simulink library "MBDS_Applications"  (R2018b)
settings: Solver=ode45  StartTime=0.0  StopTime=10.0  RelTol=1e-3
undefined symbols (not defined in the file or in its folder): Ts
libraries: KIBES_Signal x297, simulink x7
(part 6 of 6)

== system MBDS_Applications/APP_MyApplication/DTC/GetBit3/LoopOverBits ==
  note: No saturation
      | needed !
  note: Determine bit value
  note: Generate bit mask
  u : Inport
  SEL : Inport  Port=2
  Assignment1 : Assignment  IndexMode=Zero-based  IndexOptions=Index vector (port)  Indices=1  OutputSizes=[1 1]
  Bitwise Operator1 : simulink/Logic and Bit Operations/Bitwise Operator  logicop=AND  UseBitMask=off  NumInputPorts=2  BitMask=bin2dec('11011001')  BitMaskRealWorld=Stored Integer
  Constant2 : Constant  Value=0  OutDataTypeStr=Inherit: Inherit via back propagation
  Constant3 : Constant  OutDataTypeStr=Inherit: Inherit via back propagation
  Data Type Duplicate : DataTypeDuplicate  InitFcn=|
      | try
      |    MBDS_BlockCallback('Update', gcb);
      | end
  DataType : DataTypeConversion  OutDataTypeStr=boolean
  DataType1 : DataTypeConversion  OutDataTypeStr=uint8
  For Iterator : ForIterator  IterationSource=external  IndexMode=Zero-based  IterationVariableDataType=int8
  IndexOffset : Constant  Value=0  OutDataTypeStr=Inherit: Inherit via back propagation
  Relational Operator : RelationalOperator  Operator=~=  OutDataTypeStr=boolean  RndMeth=Nearest
  Selector : Selector  IndexMode=Zero-based  IndexOptions=Index vector (port)  Indices=[1 3]  OutputSizes=1
  Shift Arithmetic : ArithShift  BitShiftNumberSource=Input port  BitShiftNumber=8  BitShiftDirection=Left
      settings: InputPortMap=u0,p1
  Subtract : Sum  Inputs=+-  OutDataTypeStr=Inherit: Inherit via back propagation  InputSameDT=on
  Width : Width  DataType=uint8
  y : Outport
  wires:
  u/1 -> Data Type Duplicate/1, Bitwise Operator1/1
  DataType1/1 -> Selector/1
  SEL/1 -> Width/1, DataType/1, DataType1/1
  DataType/1 -> Assignment1/1
  Assignment1/1 -> y/1
  Relational Operator/1 -> Assignment1/2
  Constant2/1 -> Relational Operator/2
  Bitwise Operator1/1 -> Relational Operator/1
  Shift Arithmetic/1 -> Bitwise Operator1/2
  Constant3/1 -> Data Type Duplicate/2, Shift Arithmetic/1
  Width/1 -> For Iterator/1
  For Iterator/1 -> Assignment1/3, Selector/2
  Selector/1 -> Subtract/1
  Subtract/1 -> Shift Arithmetic/2
  IndexOffset/1 -> Subtract/2

== system MBDS_Applications/APP_MyApplication/DTC/GetBit4/LoopOverBits ==
  note: No saturation
      | needed !
  note: Determine bit value
  note: Generate bit mask
  u : Inport
  SEL : Inport  Port=2
  Assignment1 : Assignment  IndexMode=Zero-based  IndexOptions=Index vector (port)  Indices=1  OutputSizes=[1 1]
  Bitwise Operator1 : simulink/Logic and Bit Operations/Bitwise Operator  logicop=AND  UseBitMask=off  NumInputPorts=2  BitMask=bin2dec('11011001')  BitMaskRealWorld=Stored Integer
  Constant2 : Constant  Value=0  OutDataTypeStr=Inherit: Inherit via back propagation
  Constant3 : Constant  OutDataTypeStr=Inherit: Inherit via back propagation
  Data Type Duplicate : DataTypeDuplicate  InitFcn=|
      | try
      |    MBDS_BlockCallback('Update', gcb);
      | end
  DataType : DataTypeConversion  OutDataTypeStr=boolean
  DataType1 : DataTypeConversion  OutDataTypeStr=uint8
  For Iterator : ForIterator  IterationSource=external  IndexMode=Zero-based  IterationVariableDataType=int8
  IndexOffset : Constant  Value=0  OutDataTypeStr=Inherit: Inherit via back propagation
  Relational Operator : RelationalOperator  Operator=~=  OutDataTypeStr=boolean  RndMeth=Nearest
  Selector : Selector  IndexMode=Zero-based  IndexOptions=Index vector (port)  Indices=[1 3]  OutputSizes=1
  Shift Arithmetic : ArithShift  BitShiftNumberSource=Input port  BitShiftNumber=8  BitShiftDirection=Left
      settings: InputPortMap=u0,p1
  Subtract : Sum  Inputs=+-  OutDataTypeStr=Inherit: Inherit via back propagation  InputSameDT=on
  Width : Width  DataType=uint8
  y : Outport
  wires:
  u/1 -> Data Type Duplicate/1, Bitwise Operator1/1
  DataType1/1 -> Selector/1
  SEL/1 -> Width/1, DataType/1, DataType1/1
  DataType/1 -> Assignment1/1
  Assignment1/1 -> y/1
  Relational Operator/1 -> Assignment1/2
  Constant2/1 -> Relational Operator/2
  Bitwise Operator1/1 -> Relational Operator/1
  Shift Arithmetic/1 -> Bitwise Operator1/2
  Constant3/1 -> Data Type Duplicate/2, Shift Arithmetic/1
  Width/1 -> For Iterator/1
  For Iterator/1 -> Assignment1/3, Selector/2
  Selector/1 -> Subtract/1
  Subtract/1 -> Shift Arithmetic/2
  IndexOffset/1 -> Subtract/2

== system MBDS_Applications/APP_MyApplication/DTC/GetBit5/LoopOverBits ==
  note: No saturation
      | needed !
  note: Determine bit value
  note: Generate bit mask
  u : Inport
  SEL : Inport  Port=2
  Assignment1 : Assignment  IndexMode=Zero-based  IndexOptions=Index vector (port)  Indices=1  OutputSizes=[1 1]
  Bitwise Operator1 : simulink/Logic and Bit Operations/Bitwise Operator  logicop=AND  UseBitMask=off  NumInputPorts=2  BitMask=bin2dec('11011001')  BitMaskRealWorld=Stored Integer
  Constant2 : Constant  Value=0  OutDataTypeStr=Inherit: Inherit via back propagation
  Constant3 : Constant  OutDataTypeStr=Inherit: Inherit via back propagation
  Data Type Duplicate : DataTypeDuplicate  InitFcn=|
      | try
      |    MBDS_BlockCallback('Update', gcb);
      | end
  DataType : DataTypeConversion  OutDataTypeStr=boolean
  DataType1 : DataTypeConversion  OutDataTypeStr=uint8
  For Iterator : ForIterator  IterationSource=external  IndexMode=Zero-based  IterationVariableDataType=int8
  IndexOffset : Constant  Value=0  OutDataTypeStr=Inherit: Inherit via back propagation
  Relational Operator : RelationalOperator  Operator=~=  OutDataTypeStr=boolean  RndMeth=Nearest
  Selector : Selector  IndexMode=Zero-based  IndexOptions=Index vector (port)  Indices=[1 3]  OutputSizes=1
  Shift Arithmetic : ArithShift  BitShiftNumberSource=Input port  BitShiftNumber=8  BitShiftDirection=Left
      settings: InputPortMap=u0,p1
  Subtract : Sum  Inputs=+-  OutDataTypeStr=Inherit: Inherit via back propagation  InputSameDT=on
  Width : Width  DataType=uint8
  y : Outport
  wires:
  u/1 -> Data Type Duplicate/1, Bitwise Operator1/1
  DataType1/1 -> Selector/1
  SEL/1 -> Width/1, DataType/1, DataType1/1
  DataType/1 -> Assignment1/1
  Assignment1/1 -> y/1
  Relational Operator/1 -> Assignment1/2
  Constant2/1 -> Relational Operator/2
  Bitwise Operator1/1 -> Relational Operator/1
  Shift Arithmetic/1 -> Bitwise Operator1/2
  Constant3/1 -> Data Type Duplicate/2, Shift Arithmetic/1
  Width/1 -> For Iterator/1
  For Iterator/1 -> Assignment1/3, Selector/2
  Selector/1 -> Subtract/1
  Subtract/1 -> Shift Arithmetic/2
  IndexOffset/1 -> Subtract/2

== system MBDS_Applications/APP_MyApplication/DTC/GetBit6/LoopOverBits ==
  note: No saturation
      | needed !
  note: Determine bit value
  note: Generate bit mask
  u : Inport
  SEL : Inport  Port=2
  Assignment1 : Assignment  IndexMode=Zero-based  IndexOptions=Index vector (port)  Indices=1  OutputSizes=[1 1]
  Bitwise Operator1 : simulink/Logic and Bit Operations/Bitwise Operator  logicop=AND  UseBitMask=off  NumInputPorts=2  BitMask=bin2dec('11011001')  BitMaskRealWorld=Stored Integer
  Constant2 : Constant  Value=0  OutDataTypeStr=Inherit: Inherit via back propagation
  Constant3 : Constant  OutDataTypeStr=Inherit: Inherit via back propagation
  Data Type Duplicate : DataTypeDuplicate  InitFcn=|
      | try
      |    MBDS_BlockCallback('Update', gcb);
      | end
  DataType : DataTypeConversion  OutDataTypeStr=boolean
  DataType1 : DataTypeConversion  OutDataTypeStr=uint8
  For Iterator : ForIterator  IterationSource=external  IndexMode=Zero-based  IterationVariableDataType=int8
  IndexOffset : Constant  Value=0  OutDataTypeStr=Inherit: Inherit via back propagation
  Relational Operator : RelationalOperator  Operator=~=  OutDataTypeStr=boolean  RndMeth=Nearest
  Selector : Selector  IndexMode=Zero-based  IndexOptions=Index vector (port)  Indices=[1 3]  OutputSizes=1
  Shift Arithmetic : ArithShift  BitShiftNumberSource=Input port  BitShiftNumber=8  BitShiftDirection=Left
      settings: InputPortMap=u0,p1
  Subtract : Sum  Inputs=+-  OutDataTypeStr=Inherit: Inherit via back propagation  InputSameDT=on
  Width : Width  DataType=uint8
  y : Outport
  wires:
  u/1 -> Data Type Duplicate/1, Bitwise Operator1/1
  DataType1/1 -> Selector/1
  SEL/1 -> Width/1, DataType/1, DataType1/1
  DataType/1 -> Assignment1/1
  Assignment1/1 -> y/1
  Relational Operator/1 -> Assignment1/2
  Constant2/1 -> Relational Operator/2
  Bitwise Operator1/1 -> Relational Operator/1
  Shift Arithmetic/1 -> Bitwise Operator1/2
  Constant3/1 -> Data Type Duplicate/2, Shift Arithmetic/1
  Width/1 -> For Iterator/1
  For Iterator/1 -> Assignment1/3, Selector/2
  Selector/1 -> Subtract/1
  Subtract/1 -> Shift Arithmetic/2
  IndexOffset/1 -> Subtract/2

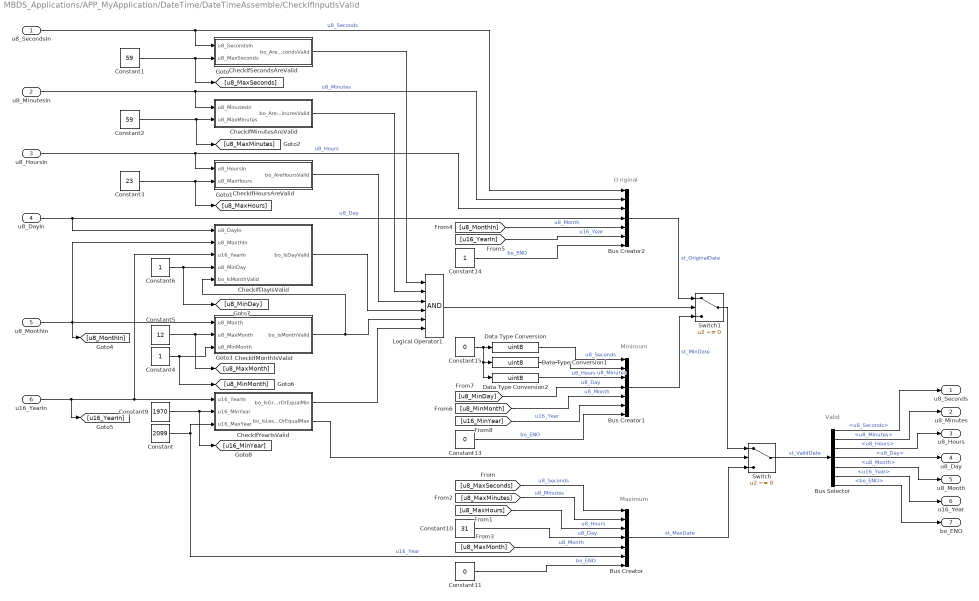
== system MBDS_Applications/APP_MyApplication/DateTime/DateTimeAssemble/CheckIfInputIsValid ==
  note: Maximum
  note: Minimum
  note: O riginal
  note: Valid
  u8_SecondsIn : Inport  OutDataTypeStr=uint8
  u8_MinutesIn : Inport  Port=2  OutDataTypeStr=uint8
  u8_HoursIn : Inport  Port=3  OutDataTypeStr=uint8
  u8_DayIn : Inport  Port=4  OutDataTypeStr=uint8
  u8_MonthIn : Inport  Port=5  OutDataTypeStr=uint8
  u16_YearIn : Inport  Port=6  OutDataTypeStr=uint16
  Bus Creator : BusCreator  Inputs='u8_Seconds','u8_Minutes','u8_Hours','u8_Day','u8_Month','u16_Year','bo_ENO'
  Bus Creator1 : BusCreator  Inputs='u8_Seconds','u8_Minutes','u8_Hours','u8_Day','u8_Month','u16_Year','bo_ENO'
  Bus Creator2 : BusCreator  Inputs='u8_Seconds','u8_Minutes','u8_Hours','u8_Day','u8_Month','u16_Year','bo_ENO'
  Bus Selector : BusSelector  OutputSignals=u8_Seconds,u8_Minutes,u8_Hours,u8_Day,u8_Month,u16_Year,bo_ENO
  CheckIfDayIsValid : Subsystem
  CheckIfHoursAreValid : Subsystem
  CheckIfMinutesAreValid : Subsystem
  CheckIfMonthIsValid : Subsystem
  CheckIfSecondsAreValid : Subsystem
  CheckIfYearIsValid : Subsystem
  Constant : Constant  Value=2099  OutDataTypeStr=uint16
  Constant1 : Constant  Value=59  OutDataTypeStr=uint8
  Constant10 : Constant  Value=31  OutDataTypeStr=uint8
  Constant11 : Constant  Value=0  OutDataTypeStr=boolean
  Constant13 : Constant  Value=0  OutDataTypeStr=boolean
  Constant14 : Constant  OutDataTypeStr=boolean
  Constant15 : Constant  Value=0  OutDataTypeStr=uint8
  Constant2 : Constant  Value=59  OutDataTypeStr=uint8
  Constant3 : Constant  Value=23  OutDataTypeStr=uint8
  Constant4 : Constant  OutDataTypeStr=uint8
  Constant5 : Constant  Value=12  OutDataTypeStr=uint8
  Constant6 : Constant  OutDataTypeStr=uint8
  Constant9 : Constant  Value=1970  OutDataTypeStr=uint16
  Data Type Conversion : DataTypeConversion  OutDataTypeStr=uint8
  Data Type Conversion1 : DataTypeConversion  OutDataTypeStr=uint8
  Data Type Conversion2 : DataTypeConversion  OutDataTypeStr=uint8
  Logical Operator1 : Logic  Inputs=6  AllPortsSameDT=off  OutDataTypeStr=boolean
  Switch : Switch  Criteria=u2 ~= 0
  Switch1 : Switch  Criteria=u2 ~= 0
  u8_Seconds : Outport  OutDataTypeStr=uint8
  u8_Minutes : Outport  Port=2  OutDataTypeStr=uint8
  u8_Hours : Outport  Port=3  OutDataTypeStr=uint8
  u8_Day : Outport  Port=4  OutDataTypeStr=uint8
  u8_Month : Outport  Port=5  OutDataTypeStr=uint8
  u16_Year : Outport  Port=6  OutDataTypeStr=uint16
  bo_ENO : Outport  Port=7  OutDataTypeStr=boolean
  wires:
  Data Type Conversion2/1 -> Bus Creator1/3  "u8_Hours"
  Data Type Conversion1/1 -> Bus Creator1/2  "u8_Minutes"
  [u16_MinYear] -> Bus Creator1/6  "u16_Year"
  Constant6/1 -> CheckIfDayIsValid/4(u8_MinDay), [u8_MinDay]
  Constant4/1 -> CheckIfMonthIsValid/3(u8_MinMonth), [u8_MinMonth]
  CheckIfYearIsValid/2(bo_IsLessOrEqualMax) -> Switch/2
  CheckIfYearIsValid/1(bo_IsGreaterOrEqualMin) -> Logical Operator1/6
  CheckIfMonthIsValid/1(bo_IsMonthValid) -> Logical Operator1/5, CheckIfDayIsValid/5(bo_IsMonthValid)
  Constant2/1 -> CheckIfMinutesAreValid/2(u8_MaxMinutes), [u8_MaxMinutes]
  CheckIfSecondsAreValid/1(bo_AreSecondsValid) -> Logical Operator1/1
  Constant1/1 -> CheckIfSecondsAreValid/2(u8_MaxSeconds), [u8_MaxSeconds]
  CheckIfDayIsValid/1(bo_IsDayValid) -> Logical Operator1/4
  u8_MonthIn/1 -> CheckIfMonthIsValid/1(u8_Month), [u8_MonthIn], CheckIfDayIsValid/2(u8_MonthIn)
  Bus Selector/5 -> u8_Month/1  "<u8_Month>"
  [u8_MaxSeconds] -> Bus Creator/1  "u8_Seconds"
  Constant15/1 -> Data Type Conversion/1, Data Type Conversion1/1, Data Type Conversion2/1
  [u8_MinDay] -> Bus Creator1/4  "u8_Day"
  Data Type Conversion/1 -> Bus Creator1/1  "u8_Seconds"
  Constant14/1 -> Bus Creator2/7  "bo_ENO"
  Switch/1 -> Bus Selector/1  "st_ValidDate"
  Bus Creator/1 -> Switch/3  "st_MaxDate"
  Switch1/1 -> Switch/1
  Bus Creator2/1 -> Switch1/1  "st_OriginalDate"
  Bus Selector/7 -> bo_ENO/1  "<bo_ENO>"
  Bus Selector/6 -> u16_Year/1  "<u16_Year>"
  Bus Selector/1 -> u8_Seconds/1  "<u8_Seconds>"
  Bus Selector/2 -> u8_Minutes/1  "<u8_Minutes>"
  Bus Selector/3 -> u8_Hours/1  "<u8_Hours>"
  Bus Selector/4 -> u8_Day/1  "<u8_Day>"
  Constant13/1 -> Bus Creator1/7  "bo_ENO"
  [u16_YearIn] -> Bus Creator2/6  "u16_Year"
  [u8_MonthIn] -> Bus Creator2/5  "u8_Month"
  Bus Creator1/1 -> Switch1/3  "st_MinDate"
  Logical Operator1/1 -> Switch1/2
  [u8_MinMonth] -> Bus Creator1/5  "u8_Month"
  [u8_MaxMonth] -> Bus Creator/5  "u8_Month"
  Constant10/1 -> Bus Creator/4  "u8_Day"
  Constant3/1 -> [u8_MaxHours], CheckIfHoursAreValid/2(u8_MaxHours)
  [u8_MaxHours] -> Bus Creator/3  "u8_Hours"
  [u8_MaxMinutes] -> Bus Creator/2  "u8_Minutes"
  Constant11/1 -> Bus Creator/7  "bo_ENO"
  Constant9/1 -> CheckIfYearIsValid/2(u16_MinYear), [u16_MinYear]
  CheckIfHoursAreValid/1(bo_AreHoursValid) -> Logical Operator1/3
  CheckIfMinutesAreValid/1(bo_AreMinutesValid) -> Logical Operator1/2
  Constant5/1 -> [u8_MaxMonth], CheckIfMonthIsValid/2(u8_MaxMonth)
  u8_DayIn/1 -> CheckIfDayIsValid/1(u8_DayIn), Bus Creator2/4  "u8_Day"
  u8_SecondsIn/1 -> Bus Creator2/1, CheckIfSecondsAreValid/1(u8_SecondsIn)  "u8_Seconds"
  u8_MinutesIn/1 -> CheckIfMinutesAreValid/1(u8_MinutesIn), Bus Creator2/2  "u8_Minutes"
  u8_HoursIn/1 -> CheckIfHoursAreValid/1(u8_HoursIn), Bus Creator2/3  "u8_Hours"
  Constant/1 -> CheckIfYearIsValid/3(u16_MaxYear), Bus Creator/6  "u16_Year"
  u16_YearIn/1 -> [u16_YearIn], CheckIfDayIsValid/3(u16_YearIn), CheckIfYearIsValid/1(u16_YearIn)

== system MBDS_Applications/APP_MyApplication/DateTime/DateTimeAssemble/ConvertToDateTime ==
  u8_Seconds : Inport  OutDataTypeStr=uint8
  u8_Minutes : Inport  Port=2  OutDataTypeStr=uint8
  u8_Hours : Inport  Port=3  OutDataTypeStr=uint8
  u16_NrOfDays : Inport  Port=4  OutDataTypeStr=uint16
  Add : Sum  Inputs=++++  OutDataTypeStr=uint32
  ConvertDaysToSeconds : Subsystem
  ConvertHoursToSeconds : Subsystem
  ConvertMinutesToSeconds : Subsystem
  u32_DateTime : Outport  OutDataTypeStr=uint32
  wires:
  u16_NrOfDays/1 -> ConvertDaysToSeconds/1(u16_NrOfDays)
  u8_Hours/1 -> ConvertHoursToSeconds/1(u8_Hours)
  u8_Minutes/1 -> ConvertMinutesToSeconds/1(u8_Minutes)
  ConvertDaysToSeconds/1(u32_SecFromDays) -> Add/4
  ConvertHoursToSeconds/1(u32_SecFromHrs) -> Add/3
  ConvertMinutesToSeconds/1(u16_SecFromMins) -> Add/2
  Add/1 -> u32_DateTime/1
  u8_Seconds/1 -> Add/1

== system MBDS_Applications/APP_MyApplication/DateTime/DateTimeAssemble/ConvertToNrOfDays ==
  note: Convert to number of days
  u8_Day : Inport  OutDataTypeStr=uint8
  u8_Month : Inport  Port=2  OutDataTypeStr=uint8
  u16_Year : Inport  Port=3  OutDataTypeStr=uint16
  AddDays : Subsystem
  AddDaysForCompleteMonths : Subsystem  TreatAsAtomicUnit=on
  AddDaysForCompleteYears : Subsystem
  CheckIfDateInLeapYearBeforeMarch : Subsystem
  Subtract2 : Sum  Inputs=+++-  OutDataTypeStr=uint16
  u16_NrOfDays : Outport  OutDataTypeStr=uint16
  wires:
  CheckIfDateInLeapYearBeforeMarch/1(bo_MinusOne) -> Subtract2/4
  AddDaysForCompleteYears/1(u16_DaysForYears) -> Subtract2/3
  AddDays/1(u8_CompleteDays) -> Subtract2/1
  AddDaysForCompleteMonths/1(u16_DaysForMonths) -> Subtract2/2
  u8_Day/1 -> AddDays/1(u8_Day)
  u8_Month/1 -> AddDaysForCompleteMonths/1(u8_Month), CheckIfDateInLeapYearBeforeMarch/1(u8_Month)
  Subtract2/1 -> u16_NrOfDays/1
  u16_Year/1 -> AddDaysForCompleteYears/1(u16_Year), CheckIfDateInLeapYearBeforeMarch/2(u16_Year)

== system MBDS_Applications/APP_MyApplication/DateTime/DateTimeDisassemble/CheckIfTimeDataIsValid ==
  note: Check if time data is valid
  note: 2099-12-31-23:59:59
  u32_DateTime : Inport  OutDataTypeStr=uint32
  Constant14 : Constant  Value=4102444799  OutDataTypeStr=uint32
  Relational Operator : RelationalOperator  Operator=<=  OutDataTypeStr=boolean  RndMeth=Nearest
  bo_ENO : Outport  OutDataTypeStr=boolean
  wires:
  Relational Operator/1 -> bo_ENO/1
  u32_DateTime/1 -> Relational Operator/1
  Constant14/1 -> Relational Operator/2

== system MBDS_Applications/APP_MyApplication/DateTime/DateTimeDisassemble/CheckLeapYearsAndRemainingDays ==
  note: avoid overflow
  note: Check leap year and calculate remaining days in current year
  note: Year
  u16_NrOfDays : Inport  OutDataTypeStr=uint16
  Add3 : Sum  Inputs=++-  OutDataTypeStr=uint16
  CalculateLeapYearsSince1970 : Subsystem
  CalculateRemainingDays : Subsystem
  CheckIfCorrectedTempYearIsLeap : Subsystem
  CheckIfTempYearIsCorrect : Subsystem
  CheckLeapYear : Subsystem
  Constant2 : Constant  OutDataTypeStr=uint16
  Constant6 : Constant  Value=0  OutDataTypeStr=uint16
  DaysPerNonLeapYear : Constant  Value=365  OutDataTypeStr=uint16
  Math Function3 : Math  Operator=rem  OutputSignalType=real  SaturateOnIntegerOverflow=on
  Relational Operator1 : RelationalOperator  Operator===  OutDataTypeStr=boolean  RndMeth=Nearest  InputSameDT=on
  Switch1 : Switch  Criteria=u2 ~= 0  OutDataTypeStr=uint16
  u16_TempDate : Outport  OutDataTypeStr=uint16
  u16_Year : Outport  Port=2  OutDataTypeStr=uint16
  bo_LeapYear : Outport  Port=3  OutDataTypeStr=boolean
  wires:
  [u16_NrOfLeapYears] -> CalculateRemainingDays/4(u16_NrOfLeapYears)
  CheckIfCorrectedTempYearIsLeap/1(bo_IsCorrectedYearLeapYear) -> CalculateRemainingDays/1(bo_IsCorrectedYearLeapYear)
  CalculateRemainingDays/1(u16_TempDate) -> u16_TempDate/1
  CheckIfTempYearIsCorrect/1(bo_IsTempYearCorrect) -> CalculateRemainingDays/2(bo_IsTempYearCorrect), Switch1/2
  [u16_NrOfLeapYears] -> CheckIfTempYearIsCorrect/2(u16_NrOfLeapYears)
  CalculateLeapYearsSince1970/1(u16_NrOfLeapYears) -> [u16_NrOfLeapYears]
  Relational Operator1/1 -> Add3/1
  Constant2/1 -> Add3/3
  Constant6/1 -> Relational Operator1/1
  CheckLeapYear/1(bo_LeapYear) -> bo_LeapYear/1
  Add3/1 -> CheckIfCorrectedTempYearIsLeap/1(u16_CorrectedTempYear), Switch1/3
  CalculateLeapYearsSince1970/2(u16_TempYear) -> Relational Operator1/2, Add3/2, Switch1/1
  Switch1/1 -> u16_Year/1, CheckLeapYear/1(u16_Year)
  Math Function3/1 -> CheckIfTempYearIsCorrect/1(u16_TempRemainingDays), CalculateRemainingDays/3(u16_TempRemainingDays)
  DaysPerNonLeapYear/1 -> CalculateLeapYearsSince1970/2(u16_DaysPerCommonYear), Math Function3/2, CalculateRemainingDays/5(u16_DaysPerCommonYear)
  u16_NrOfDays/1 -> Math Function3/1, CalculateLeapYearsSince1970/1(u16_NrOfDays)

== system MBDS_Applications/APP_MyApplication/DateTime/DateTimeDisassemble/ConvertToDayOfWeek ==
  note: Convert to day of week
  note: 1970-01-01 is Thursday
  u16_NrOfDays : Inport  OutDataTypeStr=uint16
  Add2 : Sum  OutDataTypeStr=uint16
  Add3 : Sum  OutDataTypeStr=uint16
  Constant3 : Constant  Value=7  OutDataTypeStr=uint16
  Constant4 : Constant  Value=3  OutDataTypeStr=uint8
  Constant5 : Constant  OutDataTypeStr=uint8
  Data Type Conversion3 : DataTypeConversion  OutDataTypeStr=uint8
  Math Function : Math  Operator=rem  OutputSignalType=real  SaturateOnIntegerOverflow=on
  u8_DayOfWeek : Outport  OutDataTypeStr=uint8
  wires:
  u16_NrOfDays/1 -> Add2/1
  Add3/1 -> Data Type Conversion3/1
  Math Function/1 -> Add3/1
  Add2/1 -> Math Function/1
  Constant4/1 -> Add2/2
  Constant3/1 -> Math Function/2
  Constant5/1 -> Add3/2
  Data Type Conversion3/1 -> u8_DayOfWeek/1

== system MBDS_Applications/APP_MyApplication/DateTime/DateTimeDisassemble/ConvertToMonthAndDay ==
  note: Convert to month and day
  note: Check if there are less days remaining than the next month has
  note: Count number of cycles (= Month - 1)
  note: Days per month
  u16_TempDate : Inport  OutDataTypeStr=uint16
  bo_LeapYear : Inport  Port=2  OutDataTypeStr=boolean
  Add5 : Sum  OutDataTypeStr=uint8
  CheckNrOfDaysInNextMonth : Subsystem
  Constant1 : Constant  Value=[0 31 28 31 30 31 30 31 31 30 31 30 31]  OutDataTypeStr=uint8
  Data Type Conversion : DataTypeConversion  OutDataTypeStr=uint8
  Data Type Conversion1 : DataTypeConversion  OutDataTypeStr=uint16
  Relational Operator1 : RelationalOperator  OutDataTypeStr=boolean  RndMeth=Nearest  InputSameDT=on
  SubstractDaysOfMonths : Subsystem
  Unit Delay1 : UnitDelay  SampleTime=-1
  While Iterator : WhileIterator  MaxIters=12  WhileBlockType=do-while  ResetStates=reset  ShowIterationPort=on  OutputDataType=int8
  u8_MonthMinusOne : Outport  OutDataTypeStr=uint8
  u16_DayMinusOne : Outport  Port=2  OutDataTypeStr=uint16
  wires:
  Data Type Conversion1/1 -> Relational Operator1/2
  Constant1/1 -> CheckNrOfDaysInNextMonth/1(u8_DaysPerMonth), SubstractDaysOfMonths/4(u8_DaysPerMonth)
  u16_TempDate/1 -> SubstractDaysOfMonths/1(u16_TempDate)
  CheckNrOfDaysInNextMonth/1(u8_DaysInNextMonth) -> Data Type Conversion1/1
  SubstractDaysOfMonths/1(u16_RemainingDays) -> Relational Operator1/1, u16_DayMinusOne/1
  Data Type Conversion/1 -> Add5/1
  Unit Delay1/1 -> Add5/2
  Add5/1 -> Unit Delay1/1, u8_MonthMinusOne/1
  While Iterator/1 -> CheckNrOfDaysInNextMonth/2(i8_IterationNr), SubstractDaysOfMonths/3(i8_IterationNr)
  Relational Operator1/1 -> While Iterator/1, Data Type Conversion/1
  bo_LeapYear/1 -> CheckNrOfDaysInNextMonth/3(bo_LeapYear), SubstractDaysOfMonths/2(bo_LeapYear)

== system MBDS_Applications/APP_MyApplication/DateTime/DateTimeDisassemble/ConvertToTimeAndNrOfDays ==
  note: Convert date time to time and number of days
  u32_DateTime : Inport  OutDataTypeStr=uint32
  CalculateHours : Subsystem
  CalculateMinutes : Subsystem
  CalculateSeconds : Subsystem
  u8_Seconds : Outport  OutDataTypeStr=uint8
  u8_Minutes : Outport  Port=2  OutDataTypeStr=uint8
  u8_Hours : Outport  Port=3  OutDataTypeStr=uint8
  u16_NrOfDays : Outport  Port=4  OutDataTypeStr=uint16
  wires:
  CalculateHours/1(u8_Hours) -> u8_Hours/1
  CalculateMinutes/2(u32_TempDateHrs) -> CalculateHours/1(u32_TempDateHrs)
  CalculateMinutes/1(u8_Minutes) -> u8_Minutes/1
  CalculateSeconds/2(u32_TempDateMin) -> CalculateMinutes/1(u32_TempDateMin)
  u32_DateTime/1 -> CalculateSeconds/1(u32_TimeInSeconds)
  CalculateHours/2(u16_NrOfDays) -> u16_NrOfDays/1
  CalculateSeconds/1(u8_Seconds) -> u8_Seconds/1

== system MBDS_Applications/APP_MyApplication/TimerPulse/EdgeRising/NoReset ==
  Unused1 : Inport
  Unused2 : Inport  Port=2
  u : Inport  Port=3
  Terminator : Terminator
  Terminator1 : Terminator
  y : Outport
  wires:
  Unused2/1 -> Terminator/1
  Unused1/1 -> Terminator1/1
  u/1 -> y/1

== system MBDS_Applications/APP_MyApplication/TimerPulse/Timer_RE1/DoubleReset ==
  IV : Inport
  R1 : Inport  Port=2
  R2 : Inport  Port=3
  u : Inport  Port=4
  Logical Operator : Logic  AllPortsSameDT=off  OutDataTypeStr=boolean
  Switch1 : Switch  Criteria=u2 ~= 0  OutDataTypeStr=Inherit: Inherit via back propagation  InputSameDT=on
  y : Outport
  wires:
  R2/1 -> Logical Operator/2
  R1/1 -> Logical Operator/1
  Logical Operator/1 -> Switch1/2
  IV/1 -> Switch1/1
  Switch1/1 -> y/1
  u/1 -> Switch1/3

== system MBDS_Applications/APP_MyApplication/TimerPulse/Timer_RE1/NoEnable ==
  u : Inport
  Unused1 : Inport  Port=2
  Unused2 : Inport  Port=3
  Terminator : Terminator
  Terminator1 : Terminator
  y : Outport
  wires:
  Unused1/1 -> Terminator/1
  u/1 -> y/1
  Unused2/1 -> Terminator1/1

== system MBDS_Applications/APP_MyApplication/DateTime/DateTimeAssemble/CheckIfInputIsValid/CheckIfDayIsValid ==
  note: check if day data is valid
  note: days per month
  note: Index correction
  u8_DayIn : Inport  OutDataTypeStr=uint8
  u8_MonthIn : Inport  Port=2  OutDataTypeStr=uint8
  u16_YearIn : Inport  Port=3  OutDataTypeStr=uint16
  u8_MinDay : Inport  Port=4  OutDataTypeStr=uint8
  bo_IsMonthValid : Inport  Port=5  OutDataTypeStr=boolean
  CheckIfFebruaryOfLeapYear : Subsystem
  Constant1 : Constant  OutDataTypeStr=uint8
  Constant2 : Constant  Value=[31 28 31 30 31 30 31 31 30 31 30 31]  OutDataTypeStr=uint8
  Constant20 : Constant  OutDataTypeStr=uint8
  Logical Operator1 : Logic  AllPortsSameDT=off  OutDataTypeStr=boolean
  Logical Operator3 : Logic  Operator=OR  AllPortsSameDT=off  OutDataTypeStr=boolean
  Relational Operator4 : RelationalOperator  Operator=<=  OutDataTypeStr=boolean  RndMeth=Nearest
  Relational Operator8 : RelationalOperator  OutDataTypeStr=boolean  RndMeth=Nearest
  Selector : Selector  IndexMode=Zero-based  InputPortWidth=12  IndexOptions=Index vector (port)  Indices=[1 3]  OutputSizes=1
  Subtract : Sum  Inputs=+-  OutDataTypeStr=uint8
      settings: AttributesFormatString=Saturate: %<SaturateOnIntegerOverflow>
  Switch2 : Switch  Criteria=u2 > Threshold  OutDataTypeStr=uint8
  bo_IsDayValid : Outport  OutDataTypeStr=boolean
  wires:
  Constant1/1 -> Subtract/2
  Subtract/1 -> Selector/2
  Switch2/1 -> Subtract/1
  bo_IsMonthValid/1 -> Switch2/2
  u8_MinDay/1 -> Relational Operator8/2
  CheckIfFebruaryOfLeapYear/1(bo_IsFebrauryOfLeapYear) -> Logical Operator3/2
  u8_DayIn/1 -> CheckIfFebruaryOfLeapYear/1(u8_DayIn), Relational Operator4/1, Relational Operator8/1
  Logical Operator1/1 -> bo_IsDayValid/1
  Logical Operator3/1 -> Logical Operator1/2
  Constant20/1 -> Switch2/3
  Relational Operator8/1 -> Logical Operator1/1
  Relational Operator4/1 -> Logical Operator3/1
  Selector/1 -> Relational Operator4/2
  u8_MonthIn/1 -> Switch2/1, CheckIfFebruaryOfLeapYear/2(u8_MonthIn)
  Constant2/1 -> Selector/1
  u16_YearIn/1 -> CheckIfFebruaryOfLeapYear/3(u16_YearIn)

== system MBDS_Applications/APP_MyApplication/DateTime/DateTimeAssemble/CheckIfInputIsValid/CheckIfHoursAreValid ==
  note: check if hours data is valid
  u8_HoursIn : Inport  OutDataTypeStr=uint8
  u8_MaxHours : Inport  Port=2  OutDataTypeStr=uint8
  Relational Operator3 : RelationalOperator  Operator=<=  OutDataTypeStr=boolean  RndMeth=Nearest
  bo_AreHoursValid : Outport  OutDataTypeStr=boolean
  wires:
  u8_MaxHours/1 -> Relational Operator3/2
  u8_HoursIn/1 -> Relational Operator3/1
  Relational Operator3/1 -> bo_AreHoursValid/1

== system MBDS_Applications/APP_MyApplication/DateTime/DateTimeAssemble/CheckIfInputIsValid/CheckIfMinutesAreValid ==
  note: check if minutes data is valid
  u8_MinutesIn : Inport  OutDataTypeStr=uint8
  u8_MaxMinutes : Inport  Port=2  OutDataTypeStr=uint8
  Relational Operator2 : RelationalOperator  Operator=<=  OutDataTypeStr=boolean  RndMeth=Nearest
  bo_AreMinutesValid : Outport  OutDataTypeStr=boolean
  wires:
  u8_MaxMinutes/1 -> Relational Operator2/2
  u8_MinutesIn/1 -> Relational Operator2/1
  Relational Operator2/1 -> bo_AreMinutesValid/1

== system MBDS_Applications/APP_MyApplication/DateTime/DateTimeAssemble/CheckIfInputIsValid/CheckIfMonthIsValid ==
  note: also check if month equals zero, to avoid error in 'CountDaysForCompleteMonths' Subsystem
  u8_Month : Inport  OutDataTypeStr=uint8
  u8_MaxMonth : Inport  Port=2  OutDataTypeStr=uint8
  u8_MinMonth : Inport  Port=3  OutDataTypeStr=uint8
  Logical Operator : Logic  AllPortsSameDT=off  OutDataTypeStr=boolean
  Relational Operator6 : RelationalOperator  Operator=<=  OutDataTypeStr=boolean  RndMeth=Nearest
  Relational Operator7 : RelationalOperator  OutDataTypeStr=boolean  RndMeth=Nearest
  bo_IsMonthValid : Outport  OutDataTypeStr=boolean
  wires:
  Logical Operator/1 -> bo_IsMonthValid/1
  Relational Operator7/1 -> Logical Operator/2
  Relational Operator6/1 -> Logical Operator/1
  u8_Month/1 -> Relational Operator6/1, Relational Operator7/1
  u8_MinMonth/1 -> Relational Operator7/2
  u8_MaxMonth/1 -> Relational Operator6/2

== system MBDS_Applications/APP_MyApplication/DateTime/DateTimeAssemble/CheckIfInputIsValid/CheckIfSecondsAreValid ==
  note: check if seconds data is valid
  u8_SecondsIn : Inport  OutDataTypeStr=uint8
  u8_MaxSeconds : Inport  Port=2  OutDataTypeStr=uint8
  Relational Operator : RelationalOperator  Operator=<=  OutDataTypeStr=boolean  RndMeth=Nearest
  bo_AreSecondsValid : Outport  OutDataTypeStr=boolean
  wires:
  u8_MaxSeconds/1 -> Relational Operator/2
  u8_SecondsIn/1 -> Relational Operator/1
  Relational Operator/1 -> bo_AreSecondsValid/1

== system MBDS_Applications/APP_MyApplication/DateTime/DateTimeAssemble/CheckIfInputIsValid/CheckIfYearIsValid ==
  note: check if year is less than or equal to 2099
  note: check if year is greater than or equal to 1970
  u16_YearIn : Inport  OutDataTypeStr=uint16
  u16_MinYear : Inport  Port=2  OutDataTypeStr=uint16
  u16_MaxYear : Inport  Port=3  OutDataTypeStr=uint16
  Relational Operator : RelationalOperator  OutDataTypeStr=boolean  RndMeth=Nearest
  Relational Operator1 : RelationalOperator  Operator=<=  OutDataTypeStr=boolean  RndMeth=Nearest
  bo_IsGreaterOrEqualMin : Outport  OutDataTypeStr=boolean
  bo_IsLessOrEqualMax : Outport  Port=2  OutDataTypeStr=boolean
  wires:
  Relational Operator1/1 -> bo_IsLessOrEqualMax/1
  Relational Operator/1 -> bo_IsGreaterOrEqualMin/1
  u16_MaxYear/1 -> Relational Operator1/2
  u16_MinYear/1 -> Relational Operator/2
  u16_YearIn/1 -> Relational Operator/1, Relational Operator1/1

== system MBDS_Applications/APP_MyApplication/DateTime/DateTimeAssemble/ConvertToDateTime/ConvertDaysToSeconds ==
  note: convert days to seconds
  note: 86400 sec/d
  u16_NrOfDays : Inport  OutDataTypeStr=uint16
  Constant : Constant  Value=86400  OutDataTypeStr=uint32
  Product : Product  OutDataTypeStr=uint32
  u32_SecFromDays : Outport  OutDataTypeStr=uint32
  wires:
  Product/1 -> u32_SecFromDays/1
  Constant/1 -> Product/2
  u16_NrOfDays/1 -> Product/1

== system MBDS_Applications/APP_MyApplication/DateTime/DateTimeAssemble/ConvertToDateTime/ConvertHoursToSeconds ==
  note: convert hours to seconds
  note: 3600 sec/h
  u8_Hours : Inport  OutDataTypeStr=uint8
  Constant1 : Constant  Value=3600  OutDataTypeStr=uint16
  Product1 : Product  OutDataTypeStr=uint32
  u32_SecFromHrs : Outport  OutDataTypeStr=uint32
  wires:
  Product1/1 -> u32_SecFromHrs/1
  Constant1/1 -> Product1/2
  u8_Hours/1 -> Product1/1

== system MBDS_Applications/APP_MyApplication/DateTime/DateTimeAssemble/ConvertToDateTime/ConvertMinutesToSeconds ==
  note: convert minutes to seconds
  note: 60 sec/min
  u8_Minutes : Inport  OutDataTypeStr=uint8
  Constant : Constant  Value=60  OutDataTypeStr=uint8
  Product : Product  OutDataTypeStr=uint16
  u16_SecFromMins : Outport  OutDataTypeStr=uint16
  wires:
  u8_Minutes/1 -> Product/1
  Constant/1 -> Product/2
  Product/1 -> u16_SecFromMins/1

== system MBDS_Applications/APP_MyApplication/DateTime/DateTimeAssemble/ConvertToNrOfDays/AddDays ==
  u8_Day : Inport  OutDataTypeStr=uint8
  Constant5 : Constant  OutDataTypeStr=uint8
  Subtract4 : Sum  Inputs=+-  OutDataTypeStr=uint8
  u8_CompleteDays : Outport  OutDataTypeStr=uint8
  wires:
  Subtract4/1 -> u8_CompleteDays/1
  u8_Day/1 -> Subtract4/1
  Constant5/1 -> Subtract4/2

== system MBDS_Applications/APP_MyApplication/DateTime/DateTimeAssemble/ConvertToNrOfDays/AddDaysForCompleteMonths ==
  note: add days for complete months
  u8_Month : Inport  OutDataTypeStr=uint8
  Add2 : Sum  OutDataTypeStr=uint16
  Constant1 : Constant  Value=[0 31 28 31 30 31 30 31 31 30 31 30]  OutDataTypeStr=uint8
  For Iterator : ForIterator  ResetStates=reset  IterationSource=external  IndexMode=Zero-based
  Selector : Selector  IndexMode=Zero-based  InputPortWidth=12  IndexOptions=Index vector (port)  Indices=[1 3]  OutputSizes=1
  Unit Delay1 : UnitDelay  SampleTime=-1
  u16_DaysForMonths : Outport  OutDataTypeStr=uint16
  wires:
  Add2/1 -> Unit Delay1/1, u16_DaysForMonths/1
  Unit Delay1/1 -> Add2/2
  Selector/1 -> Add2/1
  u8_Month/1 -> For Iterator/1
  For Iterator/1 -> Selector/2
  Constant1/1 -> Selector/1

== system MBDS_Applications/APP_MyApplication/DateTime/DateTimeAssemble/ConvertToNrOfDays/AddDaysForCompleteYears ==
  note: add days for complete years
  note: count leap days since 1970
  u16_Year : Inport  OutDataTypeStr=uint16
  Add : Sum  Inputs=+-  OutDataTypeStr=uint16
  Add1 : Sum  OutDataTypeStr=uint16
  Constant : Constant  Value=1970  OutDataTypeStr=uint16
  Constant1 : Constant  Value=365  OutDataTypeStr=uint16
  Constant2 : Constant  Value=1968  OutDataTypeStr=uint16
  Constant3 : Constant  Value=4  OutDataTypeStr=uint16
  Divide : Product  Inputs=*/  OutDataTypeStr=uint16
  Product : Product  OutDataTypeStr=uint16
  Subtract : Sum  Inputs=+-  OutDataTypeStr=uint16
  u16_DaysForYears : Outport  OutDataTypeStr=uint16
  wires:
  Add1/1 -> u16_DaysForYears/1
  Divide/1 -> Add1/2
  Product/1 -> Add1/1
  Constant3/1 -> Divide/2
  Subtract/1 -> Divide/1
  Constant2/1 -> Subtract/2
  Constant1/1 -> Product/2
  Add/1 -> Product/1
  Constant/1 -> Add/2
  u16_Year/1 -> Add/1, Subtract/1

== system MBDS_Applications/APP_MyApplication/DateTime/DateTimeAssemble/ConvertToNrOfDays/CheckIfDateInLeapYearBeforeMarch ==
  note: check if the date is in leap year and before the leap day
  u8_Month : Inport  OutDataTypeStr=uint8
  u16_Year : Inport  Port=2  OutDataTypeStr=uint16
  Constant2 : Constant  Value=1968  OutDataTypeStr=uint16
  Constant3 : Constant  Value=4  OutDataTypeStr=uint16
  Constant6 : Constant  Value=0  OutDataTypeStr=uint16
  Constant7 : Constant  Value=2  OutDataTypeStr=uint8
  Logical Operator : Logic  AllPortsSameDT=off  OutDataTypeStr=boolean
  Math Function : Math  Operator=rem  OutputSignalType=real  SaturateOnIntegerOverflow=on
  Relational Operator1 : RelationalOperator  Operator===  OutDataTypeStr=boolean  RndMeth=Nearest  InputSameDT=on
  Relational Operator3 : RelationalOperator  Operator=<=  OutDataTypeStr=boolean  RndMeth=Nearest
  Subtract : Sum  Inputs=+-  OutDataTypeStr=uint16
  bo_MinusOne : Outport  OutDataTypeStr=boolean
  wires:
  Logical Operator/1 -> bo_MinusOne/1
  u8_Month/1 -> Relational Operator3/1
  Relational Operator3/1 -> Logical Operator/2
  Relational Operator1/1 -> Logical Operator/1
  Constant7/1 -> Relational Operator3/2
  Constant6/1 -> Relational Operator1/2
  Math Function/1 -> Relational Operator1/1
  Constant3/1 -> Math Function/2
  Subtract/1 -> Math Function/1
  Constant2/1 -> Subtract/2
  u16_Year/1 -> Subtract/1

== system MBDS_Applications/APP_MyApplication/DateTime/DateTimeDisassemble/CheckLeapYearsAndRemainingDays/CalculateLeapYearsSince1970 ==
  u16_NrOfDays : Inport  OutDataTypeStr=uint16
  u16_DaysPerCommonYear : Inport  Port=2  OutDataTypeStr=uint16
  Add : Sum  OutDataTypeStr=uint16
  Constant : Constant  OutDataTypeStr=uint16
  Constant1 : Constant  Value=4  OutDataTypeStr=uint16
  Divide : Product  Inputs=*/  OutDataTypeStr=uint16
  Divide1 : Product  Inputs=*/  OutDataTypeStr=uint16
  u16_NrOfLeapYears : Outport  OutDataTypeStr=uint16
  u16_TempYear : Outport  Port=2  OutDataTypeStr=uint16
  wires:
  u16_DaysPerCommonYear/1 -> Divide/2
  u16_NrOfDays/1 -> Divide/1
  Divide1/1 -> u16_NrOfLeapYears/1
  Add/1 -> Divide1/1
  Constant1/1 -> Divide1/2
  Constant/1 -> Add/2
  Divide/1 -> u16_TempYear/1, Add/1

== system MBDS_Applications/APP_MyApplication/DateTime/DateTimeDisassemble/CheckLeapYearsAndRemainingDays/CalculateRemainingDays ==
  bo_IsCorrectedYearLeapYear : Inport  OutDataTypeStr=boolean
  bo_IsTempYearCorrect : Inport  Port=2  OutDataTypeStr=boolean
  u16_TempRemainingDays : Inport  Port=3  OutDataTypeStr=uint16
  u16_NrOfLeapYears : Inport  Port=4  OutDataTypeStr=uint16
  u16_DaysPerCommonYear : Inport  Port=5  OutDataTypeStr=uint16
  Add : Sum  OutDataTypeStr=uint16
  Add1 : Sum  Inputs=++-  OutDataTypeStr=uint16
  Constant : Constant  OutDataTypeStr=uint16
  Subtract : Sum  Inputs=+-  OutDataTypeStr=uint16  SaturateOnIntegerOverflow=on
      settings: AttributesFormatString=Saturate: %<SaturateOnIntegerOverflow>
  Switch : Switch  Criteria=u2 ~= 0  OutDataTypeStr=uint16
  Switch1 : Switch  Criteria=u2 ~= 0  OutDataTypeStr=uint16
  u16_TempDate : Outport  OutDataTypeStr=uint16
  wires:
  Subtract/1 -> Switch/1
  bo_IsTempYearCorrect/1 -> Switch/2
  Switch/1 -> u16_TempDate/1
  Switch1/1 -> Switch/3
  Add/1 -> Switch1/1
  Add1/1 -> Switch1/3, Add/2
  bo_IsCorrectedYearLeapYear/1 -> Switch1/2
  Constant/1 -> Add/1
  u16_DaysPerCommonYear/1 -> Add1/2
  u16_NrOfLeapYears/1 -> Subtract/2, Add1/3
  u16_TempRemainingDays/1 -> Subtract/1, Add1/1

== system MBDS_Applications/APP_MyApplication/DateTime/DateTimeDisassemble/CheckLeapYearsAndRemainingDays/CheckIfCorrectedTempYearIsLeap ==
  u16_CorrectedTempYear : Inport  OutDataTypeStr=uint16
  Add : Sum  OutDataTypeStr=uint16
  Constant : Constant  Value=2  OutDataTypeStr=uint16
  Constant1 : Constant  Value=4  OutDataTypeStr=uint16
  Constant2 : Constant  Value=0  OutDataTypeStr=uint16
  Math Function : Math  Operator=rem  OutputSignalType=real  SaturateOnIntegerOverflow=on
  Relational Operator : RelationalOperator  Operator===  OutDataTypeStr=boolean  RndMeth=Nearest
  bo_IsCorrectedYearLeapYear : Outport  OutDataTypeStr=boolean
  wires:
  Relational Operator/1 -> bo_IsCorrectedYearLeapYear/1
  Constant2/1 -> Relational Operator/2
  Constant1/1 -> Math Function/2
  Constant/1 -> Add/2
  Math Function/1 -> Relational Operator/1
  Add/1 -> Math Function/1
  u16_CorrectedTempYear/1 -> Add/1

== system MBDS_Applications/APP_MyApplication/DateTime/DateTimeDisassemble/CheckLeapYearsAndRemainingDays/CheckIfTempYearIsCorrect ==
  u16_TempRemainingDays : Inport  OutDataTypeStr=uint16
  u16_NrOfLeapYears : Inport  Port=2  OutDataTypeStr=uint16
  Relational Operator : RelationalOperator  OutDataTypeStr=boolean  RndMeth=Nearest
  bo_IsTempYearCorrect : Outport  OutDataTypeStr=boolean
  wires:
  Relational Operator/1 -> bo_IsTempYearCorrect/1
  u16_NrOfLeapYears/1 -> Relational Operator/2
  u16_TempRemainingDays/1 -> Relational Operator/1

== system MBDS_Applications/APP_MyApplication/DateTime/DateTimeDisassemble/CheckLeapYearsAndRemainingDays/CheckLeapYear ==
  note: check if the current year is a leap year
  u16_Year : Inport  OutDataTypeStr=uint16
  Add6 : Sum  OutDataTypeStr=uint16
  Constant : Constant  Value=2  OutDataTypeStr=uint8
  Constant1 : Constant  Value=4  OutDataTypeStr=uint16
  Constant9 : Constant  Value=0  OutDataTypeStr=uint16
  Math Function : Math  Operator=rem  OutputSignalType=real  SaturateOnIntegerOverflow=on
  Relational Operator2 : RelationalOperator  Operator===  OutDataTypeStr=boolean  RndMeth=Nearest  InputSameDT=on
  bo_LeapYear : Outport  OutDataTypeStr=boolean
  wires:
  Constant1/1 -> Math Function/2
  Constant/1 -> Add6/2
  Constant9/1 -> Relational Operator2/2
  Math Function/1 -> Relational Operator2/1
  u16_Year/1 -> Add6/1
  Relational Operator2/1 -> bo_LeapYear/1
  Add6/1 -> Math Function/1

== system MBDS_Applications/APP_MyApplication/DateTime/DateTimeDisassemble/ConvertToMonthAndDay/CheckNrOfDaysInNextMonth ==
  u8_DaysPerMonth : Inport  OutDataTypeStr=uint8
  i8_IterationNr : Inport  Port=2  OutDataTypeStr=int8
  bo_LeapYear : Inport  Port=3  OutDataTypeStr=boolean
  Add1 : Sum  OutDataTypeStr=uint8
  CheckNextMonthFebLeapYear : Subsystem
  Selector : Selector  IndexMode=Zero-based  InputPortWidth=13  IndexOptions=Index vector (port)  Indices=[1 3]  OutputSizes=1
  u8_DaysInNextMonth : Outport  OutDataTypeStr=uint8
  wires:
  Add1/1 -> u8_DaysInNextMonth/1
  CheckNextMonthFebLeapYear/1(bo_IsNextFebLeapYear) -> Add1/2
  Selector/1 -> Add1/1
  u8_DaysPerMonth/1 -> Selector/1
  i8_IterationNr/1 -> CheckNextMonthFebLeapYear/1(i8_IterationNr), Selector/2
  bo_LeapYear/1 -> CheckNextMonthFebLeapYear/2(bo_LeapYear)

== system MBDS_Applications/APP_MyApplication/DateTime/DateTimeDisassemble/ConvertToMonthAndDay/SubstractDaysOfMonths ==
  u16_TempDate : Inport  OutDataTypeStr=uint16
  bo_LeapYear : Inport  Port=2  OutDataTypeStr=boolean
  i8_IterationNr : Inport  Port=3  OutDataTypeStr=int8
  u8_DaysPerMonth : Inport  Port=4  OutDataTypeStr=uint8
  Add : Sum  OutDataTypeStr=uint16
  Add1 : Sum  OutDataTypeStr=uint16
  Add2 : Sum  Inputs=+-  OutDataTypeStr=uint8
  CheckCurrMonthFebLeapYear : Subsystem
  Constant : Constant  OutDataTypeStr=int8
  Selector : Selector  IndexMode=Zero-based  InputPortWidth=13  IndexOptions=Index vector (port)  Indices=[1 3]  OutputSizes=1
  Subtract : Sum  Inputs=+-  OutDataTypeStr=uint16
  Unit Delay : UnitDelay  SampleTime=-1
  u16_RemainingDays : Outport  OutDataTypeStr=uint16
  wires:
  Constant/1 -> Add2/2
  Add2/1 -> Selector/2
  Unit Delay/1 -> Add1/2
  Add1/1 -> Unit Delay/1, Subtract/2
  Add/1 -> Add1/1
  Selector/1 -> Add/2
  CheckCurrMonthFebLeapYear/1(bo_IsCurrFebLeapYear) -> Add/1
  Subtract/1 -> u16_RemainingDays/1
  u16_TempDate/1 -> Subtract/1
  u8_DaysPerMonth/1 -> Selector/1
  i8_IterationNr/1 -> CheckCurrMonthFebLeapYear/2(i8_IterationNr), Add2/1
  bo_LeapYear/1 -> CheckCurrMonthFebLeapYear/1(bo_LeapYear)

== system MBDS_Applications/APP_MyApplication/DateTime/DateTimeDisassemble/ConvertToTimeAndNrOfDays/CalculateHours ==
  note: 24 hrs/d
  u32_TempDateHrs : Inport  OutDataTypeStr=uint32
  Constant : Constant  Value=24  OutDataTypeStr=uint32
  Data Type Conversion : DataTypeConversion  OutDataTypeStr=uint8
  Data Type Conversion1 : DataTypeConversion  OutDataTypeStr=uint16
  Divide : Product  Inputs=*/  OutDataTypeStr=uint32
  Math Function : Math  Operator=rem  OutputSignalType=real  SaturateOnIntegerOverflow=on
  u8_Hours : Outport  OutDataTypeStr=uint8
  u16_NrOfDays : Outport  Port=2  OutDataTypeStr=uint16
  wires:
  u32_TempDateHrs/1 -> Math Function/1, Divide/1
  Constant/1 -> Divide/2, Math Function/2
  Data Type Conversion1/1 -> u16_NrOfDays/1
  Divide/1 -> Data Type Conversion1/1
  Data Type Conversion/1 -> u8_Hours/1
  Math Function/1 -> Data Type Conversion/1

== system MBDS_Applications/APP_MyApplication/DateTime/DateTimeDisassemble/ConvertToTimeAndNrOfDays/CalculateMinutes ==
  note: 60 min/h
  u32_TempDateMin : Inport  OutDataTypeStr=uint32
  Constant1 : Constant  Value=60  OutDataTypeStr=uint32
  Data Type Conversion1 : DataTypeConversion  OutDataTypeStr=uint8
  Divide : Product  Inputs=*/  OutDataTypeStr=uint32
  Math Function : Math  Operator=rem  OutputSignalType=real  SaturateOnIntegerOverflow=on
  u8_Minutes : Outport  OutDataTypeStr=uint8
  u32_TempDateHrs : Outport  Port=2  OutDataTypeStr=uint32
  wires:
  Data Type Conversion1/1 -> u8_Minutes/1
  Constant1/1 -> Divide/2, Math Function/2
  Divide/1 -> u32_TempDateHrs/1
  u32_TempDateMin/1 -> Math Function/1, Divide/1
  Math Function/1 -> Data Type Conversion1/1

== system MBDS_Applications/APP_MyApplication/DateTime/DateTimeDisassemble/ConvertToTimeAndNrOfDays/CalculateSeconds ==
  note: 60 sec/min
  u32_TimeInSeconds : Inport  OutDataTypeStr=uint32
  Constant : Constant  Value=60  OutDataTypeStr=uint32
  Data Type Conversion : DataTypeConversion  OutDataTypeStr=uint8
  Divide : Product  Inputs=*/  OutDataTypeStr=uint32
  Math Function : Math  Operator=rem  OutputSignalType=real  SaturateOnIntegerOverflow=on
  u8_Seconds : Outport  OutDataTypeStr=uint8
  u32_TempDateMin : Outport  Port=2  OutDataTypeStr=uint32
  wires:
  Divide/1 -> u32_TempDateMin/1
  Constant/1 -> Math Function/2, Divide/2
  Data Type Conversion/1 -> u8_Seconds/1
  Math Function/1 -> Data Type Conversion/1
  u32_TimeInSeconds/1 -> Math Function/1, Divide/1

== system MBDS_Applications/APP_MyApplication/DateTime/DateTimeAssemble/CheckIfInputIsValid/CheckIfDayIsValid/CheckIfFebruaryOfLeapYear ==
  note: check if the day is in February of a leap year
  u8_DayIn : Inport  OutDataTypeStr=uint8
  u8_MonthIn : Inport  Port=2  OutDataTypeStr=uint8
  u16_YearIn : Inport  Port=3  OutDataTypeStr=uint16
  Constant : Constant  Value=4  OutDataTypeStr=uint16
  Constant1 : Constant  Value=2  OutDataTypeStr=uint8
  Constant4 : Constant  Value=1968  OutDataTypeStr=uint16
  Constant7 : Constant  Value=29  OutDataTypeStr=uint8
  Data Type Conversion1 : DataTypeConversion  OutDataTypeStr=boolean
  Logical Operator : Logic  Inputs=3  AllPortsSameDT=off  OutDataTypeStr=boolean
  Logical Operator1 : Logic  Operator=NOT  AllPortsSameDT=off  OutDataTypeStr=boolean
  Math Function : Math  Operator=rem  OutputSignalType=real  SaturateOnIntegerOverflow=on
  Relational Operator : RelationalOperator  Operator===  OutDataTypeStr=boolean  RndMeth=Nearest
  Relational Operator1 : RelationalOperator  Operator===  OutDataTypeStr=boolean  RndMeth=Nearest
  Subtract : Sum  Inputs=+-  OutDataTypeStr=uint16  SaturateOnIntegerOverflow=on
      settings: AttributesFormatString=Saturate: %<SaturateOnIntegerOverflow>
  bo_IsFebrauryOfLeapYear : Outport  OutDataTypeStr=boolean
  wires:
  Data Type Conversion1/1 -> Logical Operator1/1
  Logical Operator/1 -> bo_IsFebrauryOfLeapYear/1
  Relational Operator/1 -> Logical Operator/2
  Constant1/1 -> Relational Operator/2
  u8_DayIn/1 -> Relational Operator1/1
  Constant/1 -> Math Function/2
  Logical Operator1/1 -> Logical Operator/3
  Math Function/1 -> Data Type Conversion1/1
  Relational Operator1/1 -> Logical Operator/1
  Constant7/1 -> Relational Operator1/2
  Subtract/1 -> Math Function/1
  Constant4/1 -> Subtract/2
  u8_MonthIn/1 -> Relational Operator/1
  u16_YearIn/1 -> Subtract/1

== system MBDS_Applications/APP_MyApplication/DateTime/DateTimeDisassemble/ConvertToMonthAndDay/CheckNrOfDaysInNextMonth/CheckNextMonthFebLeapYear ==
  note: check if next month is a February of a leap year
  i8_IterationNr : Inport  OutDataTypeStr=int8
  bo_LeapYear : Inport  Port=2  OutDataTypeStr=boolean
  Constant : Constant  Value=2  OutDataTypeStr=int8
  Logical Operator : Logic  AllPortsSameDT=off  OutDataTypeStr=boolean
  Relational Operator : RelationalOperator  Operator===  OutDataTypeStr=boolean  RndMeth=Nearest  InputSameDT=on
  bo_IsNextFebLeapYear : Outport  OutDataTypeStr=boolean
  wires:
  i8_IterationNr/1 -> Relational Operator/1
  Constant/1 -> Relational Operator/2
  bo_LeapYear/1 -> Logical Operator/2
  Relational Operator/1 -> Logical Operator/1
  Logical Operator/1 -> bo_IsNextFebLeapYear/1

== system MBDS_Applications/APP_MyApplication/DateTime/DateTimeDisassemble/ConvertToMonthAndDay/SubstractDaysOfMonths/CheckCurrMonthFebLeapYear ==
  note: check if current month is a February of a leap year
  bo_LeapYear : Inport  OutDataTypeStr=boolean
  i8_IterationNr : Inport  Port=2  OutDataTypeStr=int8
  Constant : Constant  Value=3  OutDataTypeStr=int8
  Logical Operator : Logic  AllPortsSameDT=off  OutDataTypeStr=boolean
  Relational Operator : RelationalOperator  Operator===  OutDataTypeStr=boolean  RndMeth=Nearest  InputSameDT=on
  bo_IsCurrFebLeapYear : Outport  OutDataTypeStr=boolean
  wires:
  i8_IterationNr/1 -> Relational Operator/1
  Constant/1 -> Relational Operator/2
  bo_LeapYear/1 -> Logical Operator/1
  Relational Operator/1 -> Logical Operator/2
  Logical Operator/1 -> bo_IsCurrFebLeapYear/1
